simulink model "ModulationTutorial_DSB"  (R2017a)
settings: Solver=VariableStepAuto  StartTime=0.0  StopTime=10  RelTol=1e-3
libraries: dspsrcs4 x2
settings Model: Creator=cpelabws  LastModifiedBy=cpelabws

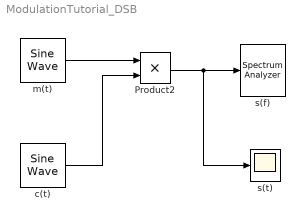
== system ModulationTutorial_DSB ==
  Product2 : Product
  c(t) : dspsrcs4/Sine Wave  Amplitude=1  Frequency=40  Phase=0  SampleMode=Discrete  OutComplex=Real  CompMethod=Trigonometric fcn  TableSize=Speed  SampleTime=1/5000  SamplesPerFrame=1  ResetState=Restart at time zero  OutputFrames=off  dataType=double  wordLen=16  udDataType=sfix(16)  fracBitsMode=Best precision  numFracBits=15  OutDataTypeStr=double  LastOutDataTypeStr=double
  m(t) : dspsrcs4/Sine Wave  Amplitude=1  Frequency=5  Phase=0  SampleMode=Discrete  OutComplex=Real  CompMethod=Trigonometric fcn  TableSize=Speed  SampleTime=1/5000  SamplesPerFrame=1  ResetState=Restart at time zero  OutputFrames=off  dataType=double  wordLen=16  udDataType=sfix(16)  fracBitsMode=Best precision  numFracBits=15  OutDataTypeStr=double  LastOutDataTypeStr=double
  s(f) : SpectrumAnalyzer
  s(t) : Scope
  wires:
  c(t)/1 -> Product2/2
  m(t)/1 -> Product2/1
  Product2/1 -> s(t)/1, s(f)/1
